simulink model "controller_2018a"  (R2018a)
settings: Solver=FixedStepAuto  StartTime=0.0  StopTime=60  FixedStep=0.1  RelTol=1e-3
settings Model: Creator=pthb3  LastModifiedBy=pthb3
settings DebuggingCC: LibraryContextMissingDiagnostic=warning
settings SFSimCC: SimUseLocalCustomCode=on
settings RTWCC: RTWUseLocalCustomCode=on

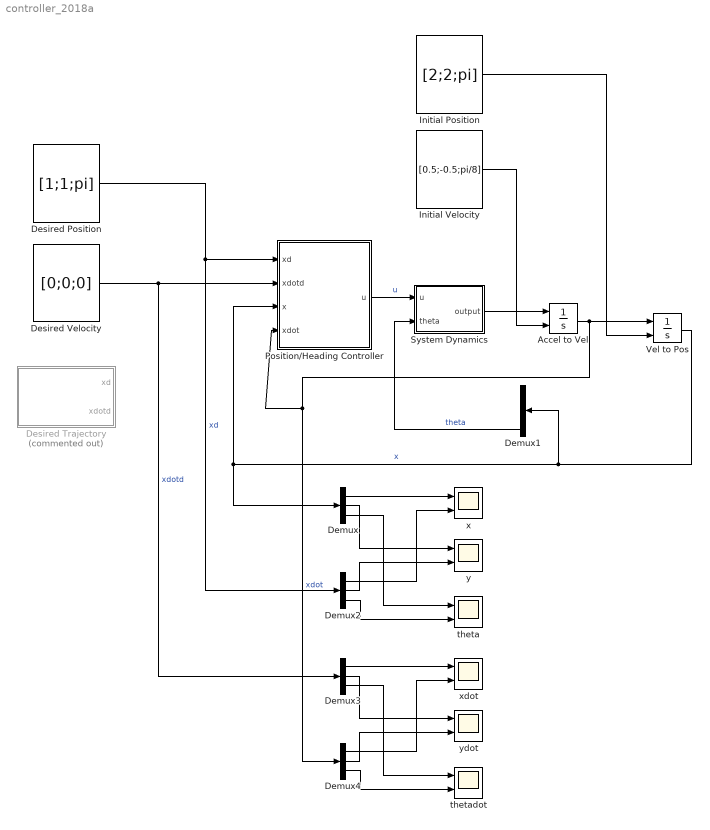
== system controller_2018a ==
  Accel to Vel : Integrator  InitialConditionSource=external  InitialCondition=[0;0;0]
  Demux{,1..4} (5 alike) : Demux  Outputs=3
  Desired Position : Constant  Value=[1;1;pi]  VectorParams1D=off
  Desired Trajectory : MATLAB Function  Commented=on  TreatAsAtomicUnit=on
  Desired Velocity : Constant  Value=[0;0;0]  VectorParams1D=off
  Initial Position : Constant  Value=[2;2;pi]  VectorParams1D=off
  Initial Velocity : Constant  Value=[0.5;-0.5;pi/8]  VectorParams1D=off
  Position/Heading Controller : MATLAB Function  TreatAsAtomicUnit=on
  System Dynamics : MATLAB Function  TreatAsAtomicUnit=on
  Vel to Pos : Integrator  InitialConditionSource=external  InitialCondition=[0;0;0]
  theta : Scope  NumInputPorts=2
  thetadot : Scope  NumInputPorts=2
  x : Scope  NumInputPorts=2
  xdot : Scope  NumInputPorts=2
  y : Scope  NumInputPorts=2
  ydot : Scope  NumInputPorts=2
  wires:
  Desired Position/1 -> Demux2/1, Position/Heading Controller/1(xd)  "xd"
  Position/Heading Controller/1(u) -> System Dynamics/1(u)  "u"
  System Dynamics/1(output) -> Accel to Vel/1
  Accel to Vel/1 -> Vel to Pos/1, Demux4/1, Position/Heading Controller/4(xdot)  "xdot"
  Vel to Pos/1 -> Demux1/1, Position/Heading Controller/3(x), Demux/1  "x"
  Desired Velocity/1 -> Demux3/1, Position/Heading Controller/2(xdotd)  "xdotd"
  Demux/1 -> x/1
  Demux/2 -> y/1
  Demux/3 -> theta/1
  Demux2/1 -> x/2
  Demux2/2 -> y/2
  Demux2/3 -> theta/2
  Demux1/3 -> System Dynamics/2(theta)  "theta"
  Demux4/3 -> thetadot/2
  Demux4/2 -> ydot/2
  Demux4/1 -> xdot/2
  Demux3/3 -> thetadot/1
  Demux3/2 -> ydot/1
  Demux3/1 -> xdot/1
  Initial Position/1 -> Vel to Pos/2
  Initial Velocity/1 -> Accel to Vel/2

== matlab function controller_2018a/Position//Heading Controller ==
  data: xd input; xdotd input; u output; x input; xdot input
function u = controller(xd,xdotd,x,xdot)

Kp = 1*eye(3);
Kd = 1*eye(3);

u = zeros(3,1);

u = (-Kd * (xdot - xdotd)) + (-Kp * (x - xd));

== matlab function controller_2018a/Desired Trajectory ==
  data: xd output; xdotd output
function [xd, xdotd]= trajectory


xd = [1,1,pi/2]';
xdotd = [0,0,0]';

== matlab function controller_2018a/System Dynamics ==
  data: u input; output output; theta input
function output  = plant(u, theta)
    L = 1;
    b = 1; 
    m = 1;
    I = 1;
    
    H = [
        -1 -1 0 0 1 1 0 0; 
        0 0 -1 -1 0 0 1 1;
        -L L -b b -L L -b b];

    T = [
        cos(theta)/m, sin(theta)/m, 0;
        -sin(theta)/m, cos(theta)/m, 0;
        0, 0, 1/(2*I)];
    
    F = H'*inv(H*H')*inv(T)*u;
    
    output = T*H*F;
end
